simulink model "GasolineEngineModel2021"  (R2021b)
settings: Solver=FixedStepAuto  StartTime=0.0  StopTime=100  FixedStep=0.05  RelTol=1e-3
libraries: simulink x1
settings Model: Creator=Combustion  LastModifiedBy=Shawn
settings DebuggingCC: UnconnectedInputMsg=none  UnconnectedOutputMsg=none  UnconnectedLineMsg=none
settings ModelReferenceCC: EnableRefExpFcnMdlSchedulingChecks=off
settings RTWCC: DLArmComputeVersion=20.02.1

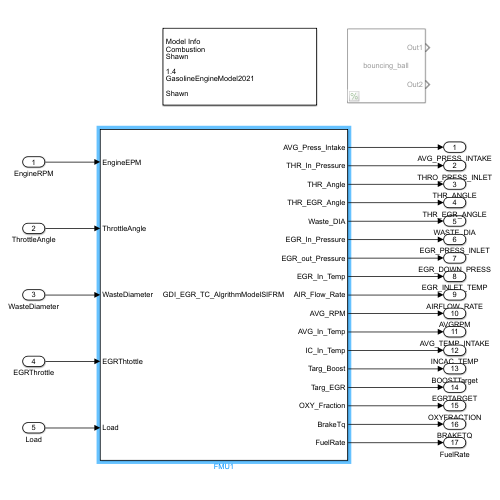
[thumbnail: Simulink's stored preview of the top-level diagram]
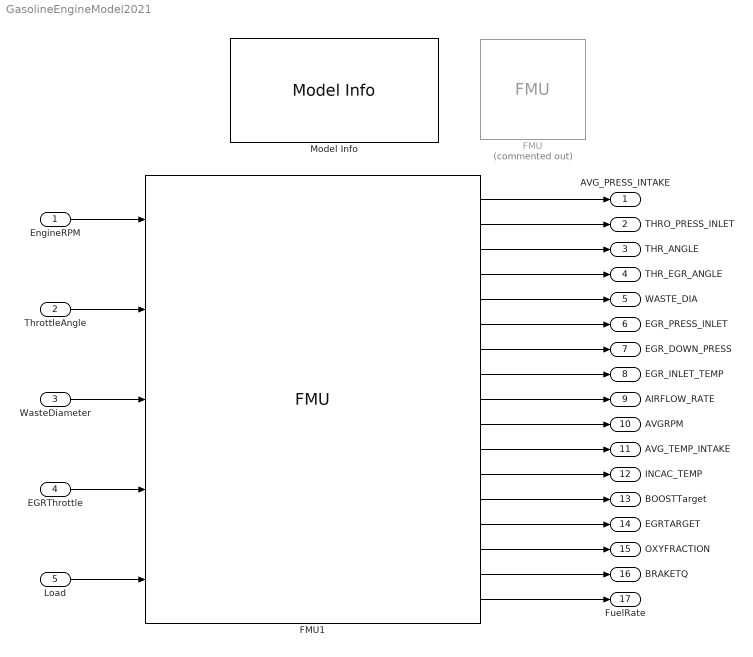
== system GasolineEngineModel2021 ==
  EngineRPM : Inport
  ThrottleAngle : Inport  Port=2
  WasteDiameter : Inport  Port=3
  EGRThrottle : Inport  Port=4
  Load : Inport  Port=5
  FMU : FMU  Commented=on  FMUName=fmuBouncingBall.fmu  FMUDebugLogging=on  FMUDebugLoggingRedirect=Display  FMUMode=ModelExchange  Param1=9.81  Param2=0.8  mask(bouncing_ball [Model Exchange, v2.0]){}
      settings: MultithreadedSim=off
      mask Display:
      | disp('bouncing_ball');
      | port_label('output',1,'Out1');
      | port_label('output',2,'Out2');
  FMU1 : FMU  FMUName=GDI_EGR_TC_AlgrithmModelSIFRM.fmu  FMUDebugLogging=on  FMUMode=CoSimulation  FMUIsToleranceUsed=on
      mask Type: GDI_EGR_TC_AlgrithmModelSIFRM [Co-Simulation, v2.0]
      mask Display:
      | disp('GDI_EGR_TC_AlgrithmModelSIFRM');
      | port_label('output',1,'AVG_Press_Intake');
      | port_label('output',2,'THR_In_Pressure');
      | port_label('output',3,'THR_Angle');
      | port_label('output',4,'THR_EGR_Angle');
      | port_label('output',5,'Waste_DIA');
      | port_label('output',6,'EGR_In_Pressure');
      | port_label('output',7,'EGR_out_Pressure');
      | port_label('output',8,'EGR_In_Temp');
      | port_label('output',9,'AIR_Flow_Rate');
      | port_label('output',10,'AVG_RPM');
      | port_label('output',11,'AVG_In_Temp');
      | port_label('output',12,'IC_In_Temp');
      | port_label('output',13,'Targ_Boost');
      | port_label('output',14,'Targ_EGR');
      | port_label('output',15,'OXY_Fraction');
      | port_label('output',16,'BrakeTq');
      | port_label('output',17,'FuelRate');
      | port_label('input',1,'EngineEPM');
      | port_label('input',2,'ThrottleAngle');
      | port_label('input',3,'WasteDiameter');
      | port_label('input',4,'EGRThtottle');
      | port_label('input',5,'Load');
  Model Info : simulink/Model-Wide Utilities/Model Info  Frame=on  DisplayStringWithTags=|  HorizontalTextAlignment=Left  LeftAlignmentValue=0.02
      | Model Info
      | %<Creator>
      | %<ModifiedBy>
      | %<ModifiedComment>
      | %<ModelVersion>
      | %<ModelName>
      | %<Description>
      | %<LastModifiedBy>
  AVG_PRESS_INTAKE : Outport
  THRO_PRESS_INLET : Outport  Port=2
  THR_ANGLE : Outport  Port=3
  THR_EGR_ANGLE : Outport  Port=4
  WASTE_DIA : Outport  Port=5
  EGR_PRESS_INLET : Outport  Port=6
  EGR_DOWN_PRESS : Outport  Port=7
  EGR_INLET_TEMP : Outport  Port=8
  AIRFLOW_RATE : Outport  Port=9
  AVGRPM : Outport  Port=10
  AVG_TEMP_INTAKE : Outport  Port=11
  INCAC_TEMP : Outport  Port=12
  BOOSTTarget : Outport  Port=13
  EGRTARGET : Outport  Port=14
  OXYFRACTION : Outport  Port=15
  BRAKETQ : Outport  Port=16
  FuelRate : Outport  Port=17
  wires:
  EngineRPM/1 -> FMU1/1
  ThrottleAngle/1 -> FMU1/2
  WasteDiameter/1 -> FMU1/3
  EGRThrottle/1 -> FMU1/4
  Load/1 -> FMU1/5
  FMU1/17 -> FuelRate/1
  FMU1/16 -> BRAKETQ/1
  FMU1/15 -> OXYFRACTION/1
  FMU1/14 -> EGRTARGET/1
  FMU1/13 -> BOOSTTarget/1
  FMU1/12 -> INCAC_TEMP/1
  FMU1/11 -> AVG_TEMP_INTAKE/1
  FMU1/10 -> AVGRPM/1
  FMU1/9 -> AIRFLOW_RATE/1
  FMU1/8 -> EGR_INLET_TEMP/1
  FMU1/7 -> EGR_DOWN_PRESS/1
  FMU1/6 -> EGR_PRESS_INLET/1
  FMU1/5 -> WASTE_DIA/1
  FMU1/4 -> THR_EGR_ANGLE/1
  FMU1/3 -> THR_ANGLE/1
  FMU1/2 -> THRO_PRESS_INLET/1
  FMU1/1 -> AVG_PRESS_INTAKE/1
